simulink model "UnitTest"  (R2020b)
settings: Solver=VariableStepAuto  StartTime=0.0  StopTime=10.0  RelTol=1e-3
libraries: simulink x3
settings Model: Creator=Mr_Li  LastModifiedBy=Mr_Li

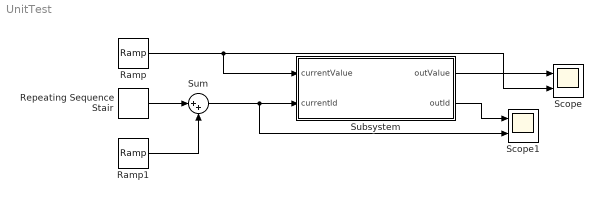
== system UnitTest ==
  Ramp : simulink/Sources/Ramp  slope=1  start=0  InitialOutput=0
  Ramp1 : simulink/Sources/Ramp  slope=1  start=0  InitialOutput=0
  Repeating Sequence Stair : simulink/Sources/Repeating Sequence Stair  OutValues=[3 1 4 2 6].'  tsamp=1  OutMin=[]  OutMax=[]  OutDataTypeStr=double  OutputDataTypeScalingMode=double  OutDataType=fixdt(0,8)  ConRadixGroup=Best Precision: Vector-wise  OutScaling=2^-12
  Scope : Scope  NumInputPorts=2
  Scope1 : Scope  NumInputPorts=2
  Subsystem : Subsystem  mask{initId=0, initValue=0}
      mask prompts: initId "Initial message ID"; initValue "Initial message value"
  Sum : Sum  Inputs=|++
  wires:
  Subsystem/1(outValue) -> Scope/1
  Ramp1/1 -> Sum/2
  Repeating Sequence Stair/1 -> Sum/1
  Sum/1 -> Scope1/2, Subsystem/2(currentId)
  Ramp/1 -> Scope/2, Subsystem/1(currentValue)
  Subsystem/2(outId) -> Scope1/1

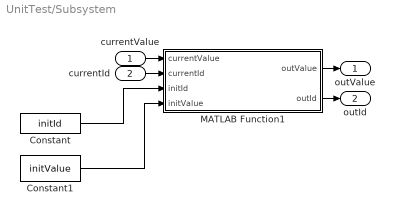
== system UnitTest/Subsystem ==
  currentValue : Inport
  currentId : Inport  Port=2
  Constant : Constant  Value=initId
  Constant1 : Constant  Value=initValue
  MATLAB Function1 : MATLAB Function  TreatAsAtomicUnit=on
  outValue : Outport
  outId : Outport  Port=2
  wires:
  MATLAB Function1/1(outValue) -> outValue/1
  currentValue/1 -> MATLAB Function1/1(currentValue)
  currentId/1 -> MATLAB Function1/2(currentId)
  MATLAB Function1/2(outId) -> outId/1
  Constant/1 -> MATLAB Function1/3(initId)
  Constant1/1 -> MATLAB Function1/4(initValue)

== matlab function UnitTest/Subsystem/MATLAB Function1 ==
  settings: updateMethod=DISCRETE
  data: currentValue input; outValue output; currentId input; initId input; initValue input; outId output
function [outValue,outId] = Buffer(currentValue,currentId,initId,initValue)

% 建立一个缓存器，根据Id来保存数据，并仅输出更新的数据

persistent bufId;
persistent bufValue;

if(isempty(bufId))
    bufId=initId;
end

if(isempty(bufValue))
    bufValue=initValue;
end

if(currentId>=bufId)
% 如果是更新的数据，更新buffer
    bufValue=currentValue;
    bufId=currentId;
end

% 直接从buffer输出
outValue=bufValue;
outId=bufId;
